simulink subsystem "PX4IO_Layer"  (R2023a)
settings: Solver=VariableStepAuto  StartTime=0.0  StopTime=10.0  RelTol=1e-3
undefined symbols (not defined in the file or in its folder): data, id, timestamp
libraries: px4uORBlib x1
settings Model: Creator=thesa  LastModifiedBy=thesa

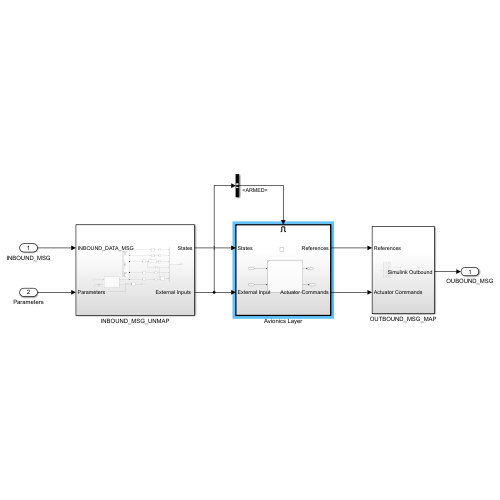
[thumbnail: Simulink's stored preview of the top-level diagram]
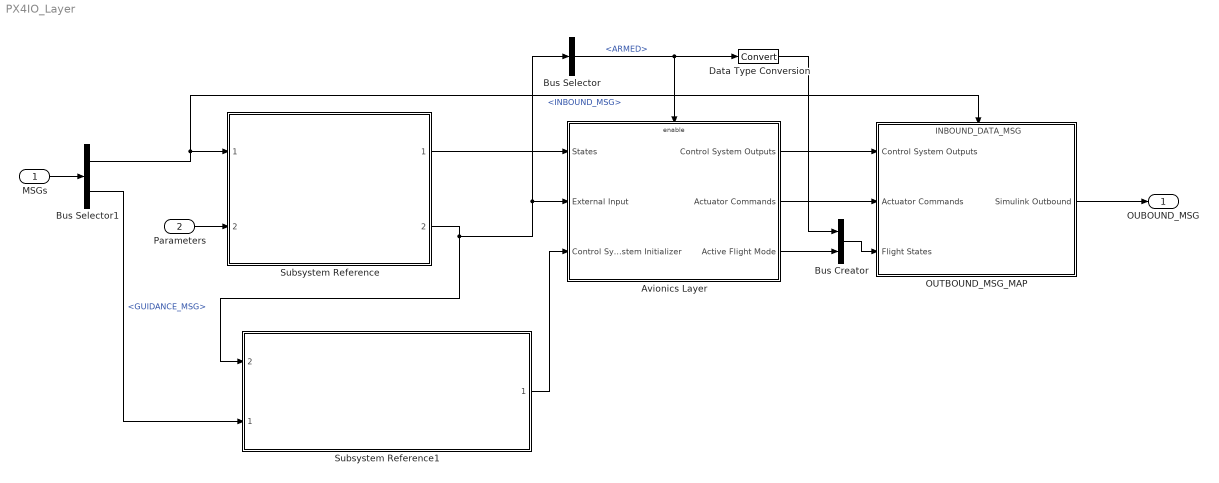
== system PX4IO_Layer ==
  MSGs : Inport
  Parameters : Inport  Port=2
  Avionics Layer : Subsystem  TreatAsAtomicUnit=on
  Bus Creator : BusCreator  Inputs=2
  Bus Selector : BusSelector  OutputSignals=Pilot Input.ARMED
  Bus Selector1 : BusSelector  OutputSignals=INBOUND_MSG,GUIDANCE_MSG
  Data Type Conversion : DataTypeConversion  SaturateOnIntegerOverflow=off  RndMeth=Floor
  OUTBOUND_MSG_MAP : Subsystem
      settings: PortSchema="{\"entries\":[{\"content\":{\"sides\":[{\"content\":{\"connectorIds\":[\"In1\",\"In2\",\"In3\"]},\"type\":\"ConnectorPlacement.EquallySpacedRectSide\",\"uuid\":\"bc4f6fb8-31ad-494c-b50f-90723c5405cd\"},{\"content\":{\"connectorIds\":[\"Out1\"],\"side\":\"RIGHT\"},\"type\":\"ConnectorPlacement.EquallySpacedRectSide\",\"uuid\":\"29e1ad7f-d8e5-4308-95be-f4da30bed432\"},{\"content\":{\"connectorIds\":[\"In4\"],\"side\":\"TOP\"},\"type\":\"ConnectorPlacement.EquallySpacedRectSide\",\"uuid\":\"033358fe-5d81-4ef8-b784-0a5a873e915b\"}]},\"type\":\"ConnectorPlacement.EquallySpacedConnector\",\"uuid\":\"616b3ee9-ff7b-4028-9ab4-30f03373fab4\"}],\"packageUris\":[\"http://schema.mathworks.com/mf0/Connector/R2020b\"],\"version\":\"1.0\"}"
  Subsystem Reference : Subsystem  ReferencedSubsystem=INBOUND_MSG_UNMAP
  Subsystem Reference1 : Subsystem  ReferencedSubsystem=GUIDANCE_MSG_UNMAP
      settings: PortSchema="{\"entries\":[{\"content\":{\"sides\":[{\"content\":{\"connectorIds\":[\"In2\",\"In1\"]},\"type\":\"ConnectorPlacement.EquallySpacedRectSide\",\"uuid\":\"d0f80337-faef-4c4a-9cc7-68c82056456e\"},{\"content\":{\"connectorIds\":[\"Out1\"],\"side\":\"RIGHT\"},\"type\":\"ConnectorPlacement.EquallySpacedRectSide\",\"uuid\":\"532281b9-6965-44c3-ba82-ea67fc3c2293\"},{\"content\":{\"side\":\"TOP\"},\"type\":\"ConnectorPlacement.EquallySpacedRectSide\",\"uuid\":\"a2424b24-61c4-4a04-b929-c29fdc2f14d0\"}]},\"type\":\"ConnectorPlacement.EquallySpacedConnector\",\"uuid\":\"dc9ea750-d322-44ba-90ee-60754d9a3045\"}],\"packageUris\":[\"http://schema.mathworks.com/mf0/Connector/R2020b\"],\"version\":\"1.0\"}"
  OUBOUND_MSG : Outport
  wires:
  Bus Selector/1 -> Data Type Conversion/1, Avionics Layer/Enable  "<ARMED>"
  Subsystem Reference/1 -> Avionics Layer/1(States)
  Bus Selector1/1 -> Subsystem Reference/1, OUTBOUND_MSG_MAP/4(INBOUND_DATA_MSG)  "<INBOUND_MSG>"
  OUTBOUND_MSG_MAP/1(Simulink Outbound) -> OUBOUND_MSG/1
  Subsystem Reference/2 -> Avionics Layer/2(External Input), Bus Selector/1, Subsystem Reference1/2
  Avionics Layer/2(Actuator Commands) -> OUTBOUND_MSG_MAP/2(Actuator Commands)
  Avionics Layer/1(Control System Outputs) -> OUTBOUND_MSG_MAP/1(Control System Outputs)
  Parameters/1 -> Subsystem Reference/2
  Avionics Layer/3(Active Flight Mode) -> Bus Creator/2
  Bus Creator/1 -> OUTBOUND_MSG_MAP/3(Flight States)
  Data Type Conversion/1 -> Bus Creator/1
  MSGs/1 -> Bus Selector1/1
  Subsystem Reference1/1 -> Avionics Layer/3(Control System Initializer)
  Bus Selector1/2 -> Subsystem Reference1/1  "<GUIDANCE_MSG>"

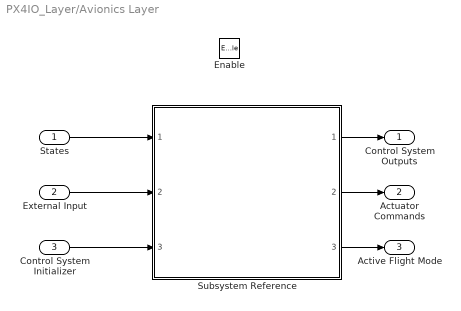
== system PX4IO_Layer/Avionics Layer ==
  States : Inport
  External Input : Inport  Port=2
  Control System Initializer : Inport  Port=3
  Enable : EnablePort  StatesWhenEnabling=reset  PropagateVarSize=During execution
  Subsystem Reference : Subsystem  ReferencedSubsystem=Controller
  Control System Outputs : Outport
  Actuator Commands : Outport  Port=2
  Active Flight Mode : Outport  Port=3
  wires:
  Control System Initializer/1 -> Subsystem Reference/3
  Subsystem Reference/3 -> Active Flight Mode/1
  External Input/1 -> Subsystem Reference/2
  States/1 -> Subsystem Reference/1
  Subsystem Reference/2 -> Actuator Commands/1
  Subsystem Reference/1 -> Control System Outputs/1

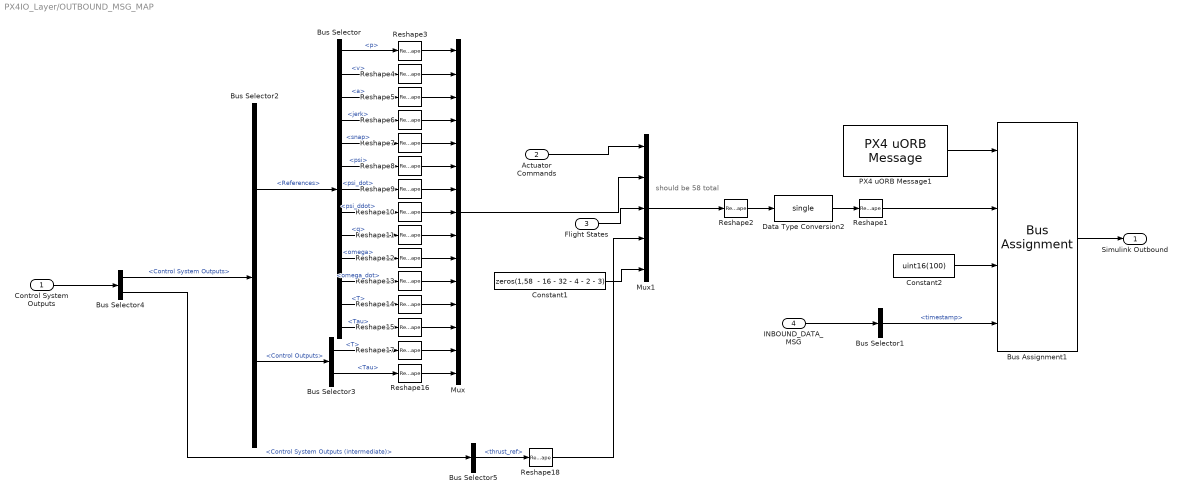
== system PX4IO_Layer/OUTBOUND_MSG_MAP ==
  note: should be 58 total
  Control System Outputs : Inport
  Actuator Commands : Inport  Port=2
  Flight States : Inport  Port=3
  INBOUND_DATA_MSG : Inport  Port=4
  Bus Assignment1 : BusAssignment  AssignedSignals=data,id,timestamp
  Bus Selector : BusSelector  OutputSignals=trajectory.p,trajectory.v,trajectory.a,trajectory.jerk,trajectory.snap,trajectory.psi,trajectory.psi_dot,trajectory.psi_ddot,reconstructed.q,reconstructed.omega,reconstructed.omega_dot,reconstructed.T,reconstructed.Tau
  Bus Selector1 : BusSelector  OutputSignals=timestamp
  Bus Selector2 : BusSelector  OutputSignals=References,Control Outputs
  Bus Selector3 : BusSelector  OutputSignals=T,Tau
  Bus Selector4 : BusSelector  OutputSignals=Control System Outputs,Control System Outputs (intermediate)
  Bus Selector5 : BusSelector  OutputSignals=thrust_ref
  Constant1 : Constant  Value="zeros(1,58  - 16 - 32 - 4 - 2 - 3)"
  Constant2 : Constant  Value=uint16(100)  OutDataTypeStr=uint16
  Data Type Conversion2 : DataTypeConversion  OutDataTypeStr=single  RndMeth=Convergent  SaturateOnIntegerOverflow=off
  Mux : Mux  Inputs=15
  Mux1 : Mux  Inputs=5
  PX4 uORB Message1 : px4uORBlib/PX4 uORB Message  uORBTopic=debug_array  SampleTime=inf  selectInstance=vehicle_gps_position
  Reshape{1..18} (18 alike) : Reshape
  Simulink Outbound : Outport
  wires:
  Reshape18/1 -> Mux1/4
  Bus Selector5/1 -> Reshape18/1  "<thrust_ref>"
  Bus Selector4/2 -> Bus Selector5/1  "<Control System Outputs (intermediate)>"
  Control System Outputs/1 -> Bus Selector4/1
  Bus Selector3/1 -> Reshape17/1  "<T>"
  Reshape17/1 -> Mux/14
  Reshape16/1 -> Mux/15
  Bus Selector3/2 -> Reshape16/1  "<Tau>"
  Bus Selector2/2 -> Bus Selector3/1  "<Control Outputs>"
  Bus Selector4/1 -> Bus Selector2/1  "<Control System Outputs>"
  Bus Selector1/1 -> Bus Assignment1/4  "<timestamp>"
  INBOUND_DATA_MSG/1 -> Bus Selector1/1
  Flight States/1 -> Mux1/3
  Mux/1 -> Mux1/2
  Bus Assignment1/1 -> Simulink Outbound/1
  Bus Selector/1 -> Reshape3/1  "<p>"
  Actuator Commands/1 -> Mux1/1
  Constant1/1 -> Mux1/5
  Bus Selector2/1 -> Bus Selector/1  "<References>"
  PX4 uORB Message1/1 -> Bus Assignment1/1
  Constant2/1 -> Bus Assignment1/3
  Reshape2/1 -> Data Type Conversion2/1
  Data Type Conversion2/1 -> Reshape1/1
  Reshape1/1 -> Bus Assignment1/2
  Mux1/1 -> Reshape2/1
  Reshape3/1 -> Mux/1
  Bus Selector/2 -> Reshape4/1  "<v>"
  Bus Selector/3 -> Reshape5/1  "<a>"
  Reshape4/1 -> Mux/2
  Reshape5/1 -> Mux/3
  Bus Selector/4 -> Reshape6/1  "<jerk>"
  Reshape6/1 -> Mux/4
  Bus Selector/5 -> Reshape7/1  "<snap>"
  Reshape7/1 -> Mux/5
  Bus Selector/6 -> Reshape8/1  "<psi>"
  Bus Selector/7 -> Reshape9/1  "<psi_dot>"
  Reshape9/1 -> Mux/7
  Reshape8/1 -> Mux/6
  Bus Selector/8 -> Reshape10/1  "<psi_ddot>"
  Reshape10/1 -> Mux/8
  Bus Selector/9 -> Reshape11/1  "<q>"
  Bus Selector/10 -> Reshape12/1  "<omega>"
  Bus Selector/11 -> Reshape13/1  "<omega_dot>"
  Bus Selector/12 -> Reshape14/1  "<T>"
  Bus Selector/13 -> Reshape15/1  "<Tau>"
  Reshape11/1 -> Mux/9
  Reshape12/1 -> Mux/10
  Reshape13/1 -> Mux/11
  Reshape14/1 -> Mux/12
  Reshape15/1 -> Mux/13
